simulink subsystem "visualization"  (R2024b)
settings: Solver=VariableStepAuto  StartTime=0.0  StopTime=10.0  RelTol=1e-3
undefined symbols (not defined in the file or in its folder): alt, angle_vert_deg, crossrange, sim_time, vel_ver
libraries: aerolibanim x1, simulink_extras x1
settings Model: Creator=joedo  LastModifiedBy=finnb

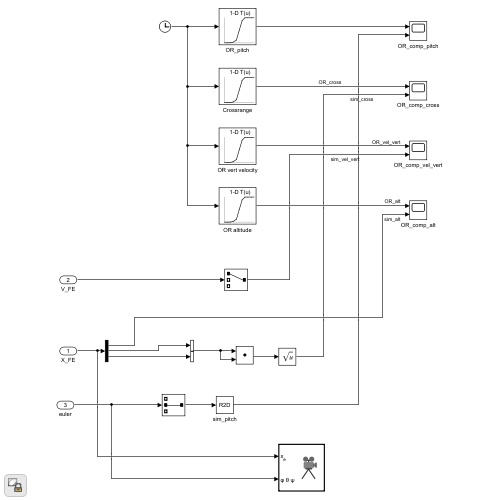
[thumbnail: Simulink's stored preview of the top-level diagram]
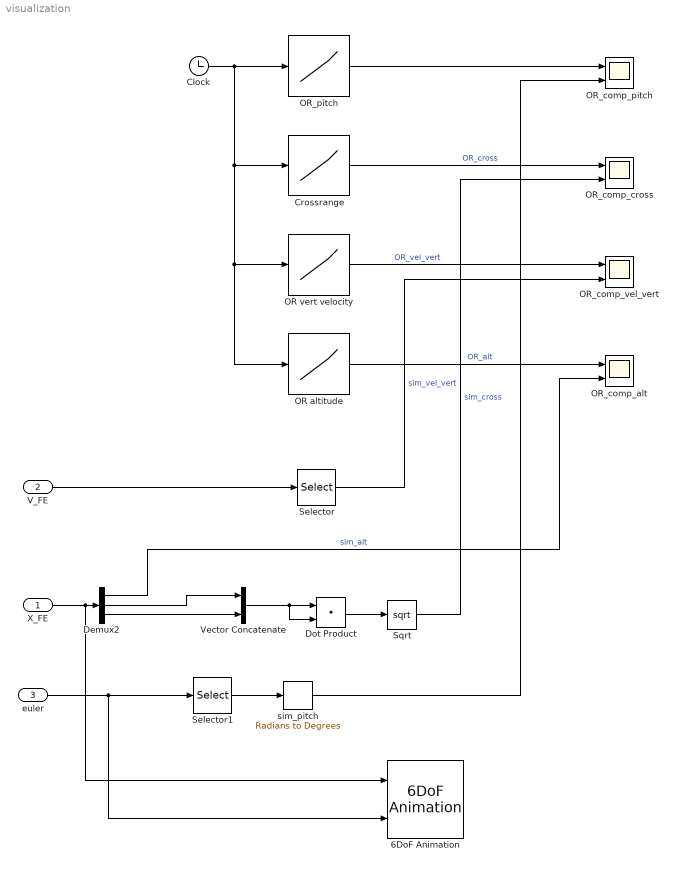
== system visualization ==
  X_FE : Inport
  V_FE : Inport  Port=2
  euler : Inport  Port=3
  6DoF Animation : aerolibanim/6DoF Animation  u1=[0 400 -200 200 0 4000]  u2=0.1  u3=100  u4=[4000 0 -5000]  u5=Fixed position  u6=[2000 500 3150]  u7=10  u8=off
  Clock : Clock
  Crossrange : Lookup_n-D  NumberOfTableDimensions=1  BreakpointsForDimension1=sim_time  Table=crossrange  InternalRulePriority=Speed  RndMeth=Simplest
  Demux2 : Demux  Outputs=3
  Dot Product : DotProduct  OutDataTypeStr=Inherit: Inherit via internal rule
  OR altitude : Lookup_n-D  NumberOfTableDimensions=1  BreakpointsForDimension1=sim_time  Table=alt  InternalRulePriority=Speed  RndMeth=Simplest
  OR vert velocity : Lookup_n-D  NumberOfTableDimensions=1  BreakpointsForDimension1=sim_time  Table=vel_ver  InternalRulePriority=Speed  RndMeth=Simplest
  OR_comp_alt : Scope  NumInputPorts=2
  OR_comp_cross : Scope  NumInputPorts=2
  OR_comp_pitch : Scope  NumInputPorts=2
  OR_comp_vel_vert : Scope  NumInputPorts=2
  OR_pitch : Lookup_n-D  NumberOfTableDimensions=1  BreakpointsForDimension1=sim_time  Table=angle_vert_deg  InternalRulePriority=Speed  RndMeth=Simplest
  Selector : Selector  InputPortWidth=3  IndexOptions=Index vector (dialog)  Indices=[1]  OutputSizes=1
  Selector1 : Selector  InputPortWidth=3  IndexOptions=Index vector (dialog)  Indices=[2]  OutputSizes=1
  Sqrt : Sqrt
  Vector Concatenate : Concatenate
  sim_pitch : simulink_extras/Transformations/Radians to Degrees
  wires:
  Vector Concatenate/1 -> Dot Product/1, Dot Product/2
  Demux2/2 -> Vector Concatenate/1
  Crossrange/1 -> OR_comp_cross/1  "OR_cross"
  Clock/1 -> OR_pitch/1, OR altitude/1, OR vert velocity/1, Crossrange/1
  Demux2/3 -> Vector Concatenate/2
  OR_pitch/1 -> OR_comp_pitch/1
  Selector1/1 -> sim_pitch/1
  sim_pitch/1 -> OR_comp_pitch/2
  OR altitude/1 -> OR_comp_alt/1  "OR_alt"
  Demux2/1 -> OR_comp_alt/2  "sim_alt"
  Selector/1 -> OR_comp_vel_vert/2  "sim_vel_vert"
  Dot Product/1 -> Sqrt/1
  Sqrt/1 -> OR_comp_cross/2  "sim_cross"
  euler/1 -> Selector1/1, 6DoF Animation/2
  OR vert velocity/1 -> OR_comp_vel_vert/1  "OR_vel_vert"
  X_FE/1 -> Demux2/1, 6DoF Animation/1
  V_FE/1 -> Selector/1
